simulink model "ModelPID"  (R2017b)
settings: Solver=FixedStepAuto  StartTime=0  StopTime=inf  RelTol=1e-3
model workspace (MAT data in the model file):
  ts = 0.1
libraries: simulink x1
settings Model: ODK_VersionTypeOld=V2.5  SimulationMode=external  Creator=Backbone  LastModifiedBy=APC_ERLF
settings DataIOCC: LimitDataPoints=on  SaveFormat=Array  SaveOutput=off  SaveTime=off
settings DebuggingCC: AllowSymbolicDim=off  SFUnexpectedBacktrackingDiag=warning  SFNoUnconditionalDefaultTransitionDiag=warning  SFExecutionAtInitializationDiag=none
settings HardwareCC: ProdBitPerPointer=32  ProdBitPerSizeT=32  ProdBitPerPtrDiffT=32  ProdWordSize=32  ProdHWDeviceType=Intel->x86-32 (Windows32)
settings ModelReferenceCC: PropagateSignalLabelsOutOfModel=off
settings RTWCC: SystemTargetFile=Target_1500S_V2_0_grt.tlc  GenCodeOnly=on  GenerateMakefile=off  TemplateMakefile=Target_1500S_V2_0_grt.tmf  Description=Target for ODK capable S7-1500 Controllers based on Simulink Coder  RTWVerbose=off  TargetLang=C++
settings CodeAppCC: ForceParamTrailComments=on  MaxIdLength=256  OperatorAnnotations=on  StateflowObjectComments=on  MATLABSourceComments=on
settings STFCustomTargetCC: ParMdlRefBuildCompliant=on  CombineOutputUpdateFcns=on  GRTInterface=off  SystemTargetFile=Target_1500S_V2_0_grt.tlc
settings GRTTargetCC: TargetLangStandard=C89/C90 (ANSI)  CompOptLevelCompliant=off  ConcurrentExecutionCompliant=off  MatFileLogging=off  CPPClassGenCompliant=off  UseToolchainInfoCompliant=off  ExtMode=on  ExtModeStaticAlloc=on  ExtModeMexFile=mwsl_ext_comm_target1500s_v2  ExtModeMexArgs='192.168.0.3'
settings ConfigComp: CovMetricSettings=dw  CovHtmlReporting=on  CovSaveCumulativeToWorkspaceVar=on  CovSaveSingleToWorkspaceVar=on  CovExternalEMLEnable=off

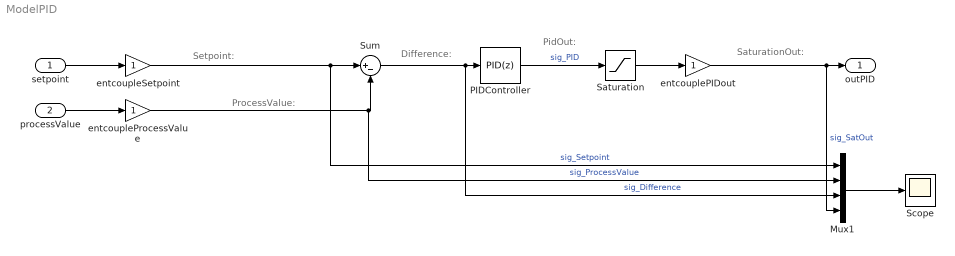
== system ModelPID ==
  note: Setpoint:
  note: ProcessValue:
  note: Difference:
  note: SaturationOut:
  note: PidOut:
  setpoint : Inport
  processValue : Inport  Port=2
  Mux1 : Mux
  PIDController : simulink/Continuous/PID Controller  Controller=PID  TimeDomain=Discrete-time  SampleTime=ts  IntegratorMethod=Forward Euler  FilterMethod=Forward Euler  Form=Parallel  UseFilter=on  ControllerParametersSource=internal  P=1.9  I=0.065  D=8.6  N=5  InitialConditionSource=internal  InitialConditionForIntegrator=0  InitialConditionForFilter=0  ExternalReset=none  LimitOutput=off  UpperSaturationLimit=100  LowerSaturationLimit=0.0  LinearizeAsGain=off  AntiWindupMode=clamping  Kb=1  TrackingMode=off  Kt=1  PParamMin=[]  PParamMax=[]  IParamMin=[]  IParamMax=[]  DParamMin=[]  DParamMax=[]  NParamMin=[]  NParamMax=[]  KbParamMin=[]  KbParamMax=[]  KtParamMin=[]  KtParamMax=[]  POutMin=[]  POutMax=[]  IOutMin=[]  IOutMax=[]  DOutMin=[]  DOutMax=[]  DOutDataTypeStr=double  DGainOutDataTypeStr=double  DProdOutDataTypeStr=double  NOutMin=[]  NOutMax=[]  KbOutMin=[]  KbOutMax=[]  KtOutMin=[]  KtOutMax=[]  IntegratorOutMin=[]  IntegratorOutMax=[]  FilterOutMin=[]  FilterOutMax=[]  SumOutMin=[]  SumOutMax=[]  SumI1OutMin=[]  SumI1OutMax=[]  SumI2OutMin=[]  SumI2OutMax=[]  SumI3OutMin=[]  SumI3OutMax=[]  SumDOutMin=[]  SumDOutMax=[]  SaturationOutMin=[]  SaturationOutMax=[]  IntegratorContinuousStateAttributes=''  IntegratorStateMustResolveToSignalObject=off  IntegratorRTWStateStorageClass=Auto  FilterContinuousStateAttributes=''  FilterStateMustResolveToSignalObject=off  FilterRTWStateStorageClass=Auto  DifferentiatorICPrevScaledInput=0  DifferentiatorOutMin=[]  DifferentiatorOutMax=[]  InitialConditionSetting=State (most efficient)  FilterDiffOutCoefMin=[]  FilterDiffOutCoefMax=[]  SumDenOutMin=[]  SumDenOutMax=[]  SumNumOutMin=[]  SumNumOutMax=[]  ReciprocalOutMin=[]  ReciprocalOutMax=[]  DivideOutMin=[]  DivideOutMax=[]  TunerSelectOption=Transfer Function Based (PID Tuner App)
  Saturation : Saturate  UpperLimit=100  LowerLimit=0
  Scope : Scope
  Sum : Sum  Inputs=|+-
  entcouplePIDout : Gain
  entcoupleProcessValue : Gain
  entcoupleSetpoint : Gain
  outPID : Outport
  wires:
  Sum/1 -> Mux1/3, PIDController/1  "sig_Difference"
  setpoint/1 -> entcoupleSetpoint/1
  entcoupleSetpoint/1 -> Mux1/1, Sum/1  "sig_Setpoint"
  processValue/1 -> entcoupleProcessValue/1
  entcoupleProcessValue/1 -> Mux1/2, Sum/2  "sig_ProcessValue"
  Mux1/1 -> Scope/1
  PIDController/1 -> Saturation/1  "sig_PID"
  entcouplePIDout/1 -> Mux1/4, outPID/1  "sig_SatOut"
  Saturation/1 -> entcouplePIDout/1
